simulink model "Feedback_diversity"  (R2023b)
settings: Solver=VariableStepAuto  StartTime=0.0  StopTime=10.0  RelTol=1e-3
undefined symbols (not defined in the file): DiscIntNeverNeededParam, doppler
libraries: commchan3 x2, commdigbbndpm3 x2
settings Model: Creator=hema2  LastModifiedBy=hema2

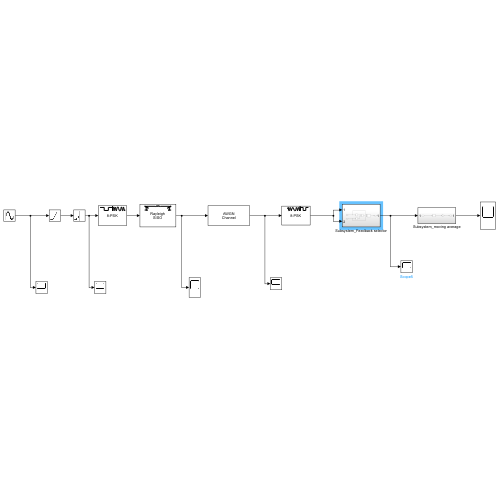
[thumbnail: Simulink's stored preview of the top-level diagram]
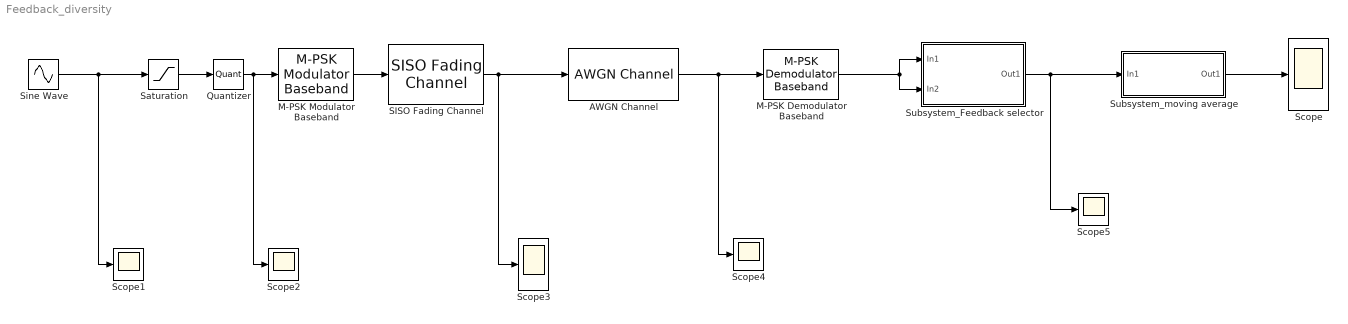
== system Feedback_diversity ==
  AWGN Channel : commchan3/AWGN Channel  LegacyMode=off  NoiseMethod="Signal to noise ratio  (Eb/No)"  noiseMode="Signal to noise ratio  (SNR)"  EbNo=10  EsNo=10  SNR=8  BitsPerSymbol=3  SignalPower=1  SamplesPerSymbol=1  SymbolPeriod=1  VarianceSource=Parameter  Variance=1  RandomStream=Global stream  Seed=67  SimulateUsing=Code generation
  M-PSK Demodulator Baseband : commdigbbndpm3/M-PSK Demodulator Baseband  M=8  OutType=Integer  DecType=Hard decision  VarSource=Dialog  Variance=1  Dec=Gray  Mapping=[0:7]  Ph=0  outDtype1=Inherit via internal rule  outDtype2=Inherit via internal rule  derotateFactorWordLen=16  derotateFactorDataTypeStr=Inherit: Same word length as input  derotateFactorLastDataTypeStr=Inherit: Same word length as input
  M-PSK Modulator Baseband : commdigbbndpm3/M-PSK Modulator Baseband  M=8  InType=Integer  Enc=Gray  Mapping=[0:7]  Ph=pi/8  outDtype=double  outWordLen=16  outUDDataType=sfix(16)  outFracLenMode=Best precision  outFracLen=15  outDataTypeStr=double  outLastDataTypeStr=double
  Quantizer : Quantizer  QuantizationInterval=1
  SISO Fading Channel : commchan3/SISO Fading Channel  InheritSampleRate=on  SampleRate=1000000  PathDelays=[0 1.5e-5]  AveragePathGains=[0 -3]  NormalizePathGains=on  FadingDistribution=Rayleigh  KFactor=3  DirectPathDopplerShift=0  DirectPathInitialPhase=0  MaximumDopplerShift=10  DopplerSpectrum=doppler('Jakes')  RandomStream=mt19937ar with seed  Seed=73  PathGainsOutputPort=off  ChannelFilterDelayOutputPort=off  SimulateUsing=Interpreted execution  Visualization=Off  PathsForDopplerDisplay=1  SamplesToDisplay=25%
  Saturation : Saturate  UpperLimit=7  LowerLimit=0
  Scope{,1..5} (6 alike) : Scope
  Sine Wave : Sin  Amplitude=3  Frequency=1000000  SampleTime=1/1000000
  Subsystem_Feedback selector : Subsystem
  Subsystem_moving average : Subsystem
  wires:
  AWGN Channel/1 -> Scope4/1, M-PSK Demodulator Baseband/1
  M-PSK Modulator Baseband/1 -> SISO Fading Channel/1
  SISO Fading Channel/1 -> Scope3/1, AWGN Channel/1
  Subsystem_moving average/1(Out1) -> Scope/1
  Subsystem_Feedback selector/1(Out1) -> Subsystem_moving average/1(In1), Scope5/1
  M-PSK Demodulator Baseband/1 -> Subsystem_Feedback selector/2(In2), Subsystem_Feedback selector/1(In1)
  Saturation/1 -> Quantizer/1
  Quantizer/1 -> Scope2/1, M-PSK Modulator Baseband/1
  Sine Wave/1 -> Scope1/1, Saturation/1

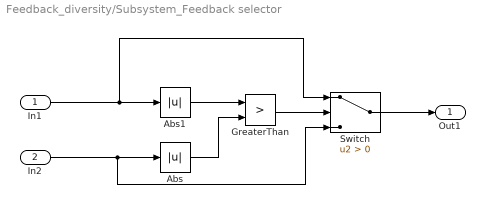
== system Feedback_diversity/Subsystem_Feedback selector ==
  In1 : Inport
  In2 : Inport  Port=2
  Abs : Abs  SaturateOnIntegerOverflow=off
  Abs1 : Abs  SaturateOnIntegerOverflow=off
  GreaterThan : RelationalOperator  Operator=>  OutDataTypeStr=boolean  RndMeth=Simplest  InputSameDT=off
  Switch : Switch  Criteria=u2 > Threshold  SaturateOnIntegerOverflow=off  InputSameDT=off
  Out1 : Outport
  wires:
  Switch/1 -> Out1/1
  Abs1/1 -> GreaterThan/1
  In2/1 -> Switch/3, Abs/1
  Abs/1 -> GreaterThan/2
  In1/1 -> Switch/1, Abs1/1
  GreaterThan/1 -> Switch/2

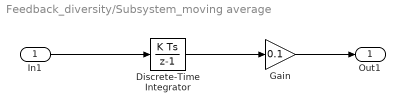
== system Feedback_diversity/Subsystem_moving average ==
  In1 : Inport
  Discrete-Time Integrator : DiscreteIntegrator  SampleTime=-1  ICPrevOutput=DiscIntNeverNeededParam  ICPrevScaledInput=DiscIntNeverNeededParam
  Gain : Gain  Gain=0.1
  Out1 : Outport
  wires:
  In1/1 -> Discrete-Time Integrator/1
  Discrete-Time Integrator/1 -> Gain/1
  Gain/1 -> Out1/1
